simulink subsystem "PID_gain_scheduling"  (R2024a)
settings: Solver=VariableStepAuto  StartTime=0.0  StopTime=10.0  RelTol=1e-3
values from neighbouring files (symbols this model uses):
  PID = pid(-125, -377.830, -5.65)    [PID_design.m]
undefined symbols (not defined in the file or in its folder): u_eq
settings Model: Creator=Bocchio  LastModifiedBy=Bocchio

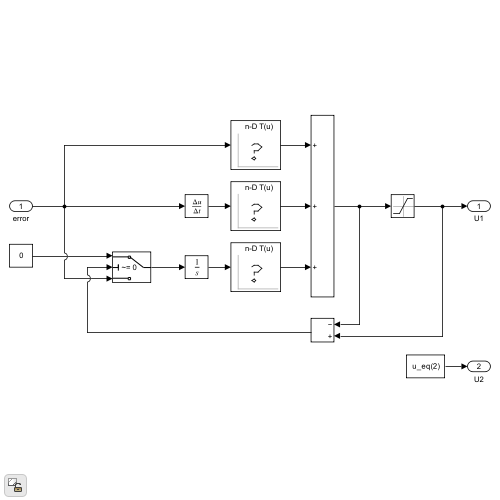
[thumbnail: Simulink's stored preview of the top-level diagram]
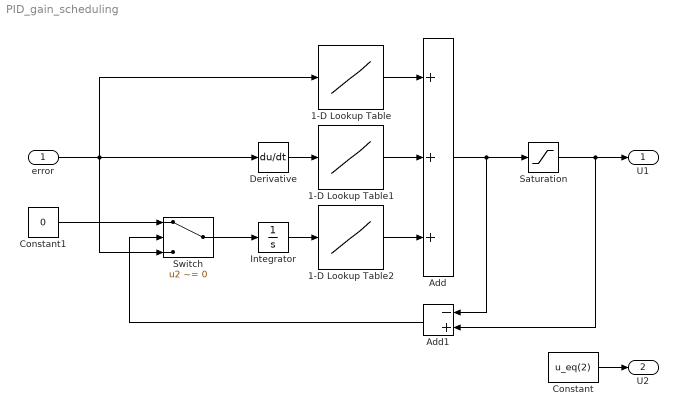
== system PID_gain_scheduling ==
  error : Inport
  1-D Lookup Table : Lookup_n-D  NumberOfTableDimensions=1  BreakpointsForDimension1=[-5:5]  Table=PID.Kp  InternalRulePriority=Speed  RndMeth=Simplest
  1-D Lookup Table1 : Lookup_n-D  NumberOfTableDimensions=1  BreakpointsForDimension1=[-5:5]  Table=PID.Kd  InternalRulePriority=Speed  RndMeth=Simplest
  1-D Lookup Table2 : Lookup_n-D  NumberOfTableDimensions=1  BreakpointsForDimension1=[-5:5]  Table=PID.Ki  InternalRulePriority=Speed  RndMeth=Simplest
  Add : Sum  Inputs=+++
  Add1 : Sum  Inputs=-+
  Constant : Constant  Value=u_eq(2)
  Constant1 : Constant  Value=0
  Derivative : Derivative  CoefficientInTFapproximation=1e6
  Integrator : Integrator
  Saturation : Saturate  UpperLimit=1  LowerLimit=0
  Switch : Switch  Criteria=u2 ~= 0  SaturateOnIntegerOverflow=off  InputSameDT=off
  U1 : Outport
  U2 : Outport  Port=2
  wires:
  Constant/1 -> U2/1
  error/1 -> Derivative/1, 1-D Lookup Table/1, Switch/3
  1-D Lookup Table2/1 -> Add/3
  Derivative/1 -> 1-D Lookup Table1/1
  Add/1 -> Saturation/1, Add1/1
  1-D Lookup Table1/1 -> Add/2
  Switch/1 -> Integrator/1
  Add1/1 -> Switch/2
  1-D Lookup Table/1 -> Add/1
  Saturation/1 -> Add1/2, U1/1
  Constant1/1 -> Switch/1
  Integrator/1 -> 1-D Lookup Table2/1
